simulink model "AdvancedLabModel"  (R2023a)
settings: Solver=ode45  StartTime=0.0  StopTime=10  RelTol=1e-3
settings Model: Creator=mazen  LastModifiedBy=mazen

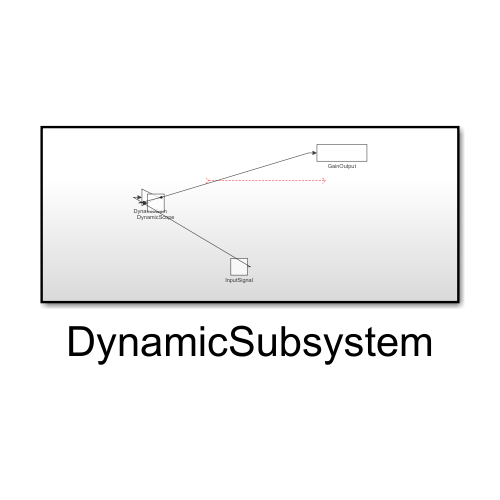
[thumbnail: Simulink's stored preview of the top-level diagram]
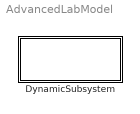
== system AdvancedLabModel ==
  DynamicSubsystem : Subsystem

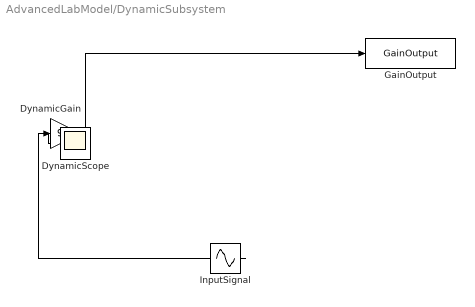
== system AdvancedLabModel/DynamicSubsystem ==
  DynamicGain : Gain  Gain=9
  DynamicScope : Scope
  GainOutput : ToWorkspace  VariableName=GainOutput  SaveFormat=Structure With Time  SampleTime=-1
  InputSignal : Sin  SampleTime=0
  wires:
  ? -> ?
  InputSignal/1 -> DynamicGain/1
  DynamicGain/1 -> DynamicScope/1, GainOutput/1
